simulink model "DemonstratorSimscape_GMM1"  (R2021b)
settings: Solver=ode113  StartTime=0.0  StopTime=t_stop*0+20  FixedStep=1e-4
values from neighbouring files (symbols this model uses):
  brkD = 0    [main.m]
  brkI = 1e4    (= 10000)    [main.m]
  brkP = 1e5    (= 100000)    [main.m]
  d_drm = 0.5*d_drum    [main.m]
  d_shm = 0.4*d_sheave    [main.m]
  DeltaCable0 = 0    [main.m]
  Droop_scaling = 0    [main.m]
  eta_sh = 0.015    [main.m]
  filt_NUM = ones(1,200)*0.005    [main.m]
  g = 9.80665    [main.m]
  Iw = 0.5*(W.i + M.in*GB.r^2)    [main.m]
  Kp_mul = 0.3    [main.m]
  Lc0 = abs((T.ph-L.height-P.d-L.z0)*0.001)    [main.m]
  Ls1 = ((T.ph-0.5*W.pd)/1000)    [main.m]
  Ls2 = ((0.5*(T.s2+P.d)-2*P.d)/1000)    [main.m]
  M = 50e3    (= 50000)    [calcGrav.m]
  phi0_drm = -90    [main.m]
  phi0_shm = -90    [main.m]
  r_sheave = P.d*0.5    [main.m]
  s = tf('s')    [calcGrav.m]
  tau_brk = 0.001    [main.m]
  tau_em = 60e-3    (= 0.06)    [calcGrav.m]    (also in main.m)
  tau_m = tau_w/GB.r    [main.m]
  Tmax = 400e3    (= 400000)    [main.m]
  Tn_mul = 10    [main.m]
  x_drm = 0.7*r_drum    [main.m]
  x_shm = 0.7*r_sheave    [main.m]
  z0 = 0    [calcGrav.m]    (also in main.m = L.z0-P.d*0.5-P.d-P.d-L.height-T.h1-T.h2-32)
undefined symbols (not defined in the file or in its folder): C, CA, Controller_sampleTime, DiscIntNeverNeededParam, GB, L, P, Part, T, VFD_acceleration_model_factor, VFD_Adapt_factor_lower_p1458, VFD_Adapt_factor_upper_p1459, VFD_Curr_limit_var_p0641, VFD_Current_limit_p0640, VFD_Id_setp_total_r1624, VFD_Iq, VFD_Kp_n_basic_p1460, VFD_M, VFD_M_accel_T_smooth_p1517, VFD_M_lim_var_fixS_src_p1551, VFD_M_max_lower_p1521, VFD_M_max_lower_scal_p1525, VFD_M_max_up_mot_scal_p1524, VFD_M_max_upper_p1520, VFD_n_act_T_smooth_p1442, VFD_n_ctr_Kp_n_up_scal_p1461, VFD_n_ctr_Tn_n_up_sca_p1463, VFD_n_ctrl_adapt_Kp_lower_p1456, VFD_n_ctrl_adapt_Kp_upper_p1457, VFD_n_ctrl_Adpt_sig_Kp_p1455, VFD_n_ctrl_Kp_scal_p1466, VFD_n_ctrl_n_lower_p1464, VFD_n_ctrl_n_upper_p1465, VFD_n_ctrl_Tn_n_lower_p1462, VFD_n_limit_neg_p1086, VFD_n_limit_pos_p1083, VFD_n_limit_setp_p1063, VFD_n_max_p1082, VFD_n_set_filt_1_T_p1416, VFD_P_max_gen_p1531, VFD_P_max_mot_p1530, VFD_PU_I_outp_max_r0289, VFD_RFG_ramp_down_time_p1121, VFD_RFG_ramp_up_time_p1120, VFD_RFG_t_RD_scal_p1139, VFD_RFG_t_RU_scal_p1138, VSD, W, X, Y, Z
libraries: sm_lib x248, nesl_utility x128, simulink x49, cstblocks x2, pid_lib x2, slpidlib x2, simulink_extras x2
(part 5 of 11)

== system DemonstratorSimscape_GMM1/Transmission System/Anchor and Load/Sheave_05 ==
  Bending loss : Subsystem  Commented=on
  Gain : Gain  Gain=-1
  Nm : nesl_utility/Simulink-PS Converter  PhysicalDomain=network_engine_domain  SubClassName=ps_input  LeftPortType=input  RightPortType=output  PseudoPeriodic=off  Frequencies=[]  NoiseDistribution=none  NoiseParameters=[]  Unit=1  AffineConversion=off  FilteringAndDerivatives=filter  SimscapeFilterOrder=2  InputFilterTimeConstant=tau_bending  UdotUserProvided=0
      settings: SourceProductBaseCode=PW,SS
  PS>Sim2 : Subsystem
  Pulley 5 : sm_lib/Belts and Cables/Pulley  PitchRadius=P.d*0.5  PitchRadiusUnits=mm  InitialWrapAngleLowerBound=0.0  InitialWrapAngleLowerBoundUnits=deg  SenseWrapAngle=off  SensePulleyAngleA=off  SensePulleyAngleB=off  SenseFleetAngleA=off  SenseFleetAngleB=off
      settings: SourceProductBaseCode=MS
  Revolute Pulley5 : sm_lib/Joints/Revolute Joint  JointMode=Normal  SenseConstraintForce=on  SenseConstraintForceX=off  SenseConstraintForceY=off  SenseConstraintForceZ=off  SenseConstraintTorque=on  SenseConstraintTorqueX=off  SenseConstraintTorqueY=off  SenseConstraintTorqueZ=off  SenseTotalForce=on  SenseTotalForceX=off  SenseTotalForceY=off  SenseTotalForceZ=off  SenseTotalTorque=on  SenseTotalTorqueX=off  SenseTotalTorqueY=off  SenseTotalTorqueZ=off  CompositeWrenchDir=FollowerOnBase  CompositeWrenchFrame=BaseFrame  EquilibriumPosition=0  EquilibriumPositionUnits=deg  SpringStiffness=0  SpringStiffnessUnits=N*m/deg  DampingCoefficient=b_pulley  DampingCoefficientUnits=N*m/(deg/s)  TorqueActuationMode=InputTorque  MotionActuationMode=ComputedMotion  SensePosition=on  SenseVelocity=on  SenseAcceleration=on  SenseTorqueForce=on  SenseLowerLimitTorqueForce=off  SenseUpperLimitTorqueForce=off  LowerLimitSpecify=off  LowerLimitBound=-90  LowerLimitBoundUnits=deg  LowerLimitStiffness=1e4  LowerLimitStiffnessUnits=N*m/deg  LowerLimitDamping=10  LowerLimitDampingUnits=N*m/(deg/s)  LowerLimitTransitionRegionWidth=0.1  LowerLimitTransitionRegionWidthUnits=deg  UpperLimitSpecify=off  UpperLimitBound=90  UpperLimitBoundUnits=deg  UpperLimitStiffness=1e4  UpperLimitStiffnessUnits=N*m/deg  UpperLimitDamping=10  UpperLimitDampingUnits=N*m/(deg/s)  UpperLimitTransitionRegionWidth=0.1  UpperLimitTransitionRegionWidthUnits=deg  PositionTargetSpecify=off  PositionTargetPriority=High  PositionTargetValue=0  PositionTargetValueUnits=deg  VelocityTargetSpecify=off  VelocityTargetPriority=High  VelocityTargetValue=0  VelocityTargetValueUnits=deg/s
  ScopePulley5 : Scope  Commented=on  NumInputPorts=8
  Sheave5 : Subsystem
      mask Display: image('sm_cable_drive_right_angle_pulleyA_IMAGE.png');
  w (rad/s)1 : nesl_utility/PS-Simulink Converter  PhysicalDomain=network_engine_domain  SubClassName=ps_output  LeftPortType=input  RightPortType=output  PseudoPeriodic=off  Frequencies=[]  Unit=rad/s  AffineConversion=on
      settings: SourceProductBaseCode=PW,SS
  ConnS5 : PMIOPort  Side=Right
  WireA : PMIOPort  Port=2  Side=Left
  WireB : PMIOPort  Port=3  Side=Left
  w (rad/s) : Outport
  tag scope: S4=global, w5=global
  wires:
  PS>Sim2/6(Out6) -> ScopePulley5/6
  PS>Sim2/3(Out3) -> ScopePulley5/3
  PS>Sim2/4(Out4) -> ScopePulley5/4
  PS>Sim2/7(Out7) -> ScopePulley5/7
  PS>Sim2/1(Out1) -> ScopePulley5/1
  PS>Sim2/5(Out5) -> ScopePulley5/5
  PS>Sim2/2(Out2) -> ScopePulley5/2
  PS>Sim2/8(Out8) -> ScopePulley5/8
  w (rad/s)1/1 -> Gain/1, w (rad/s)/1
  [S5] -> Bending loss/1(Sin (kN))
  Bending loss/1(dT (Nm)) -> Nm/1
  Bending loss/2(Sout (kN)) -> [S4]
  Gain/1 -> [w5], Bending loss/2(w (deg/s))
  connections:
  w (rad/s)1/LConn1 -- Revolute Pulley5/RConn3 -- PS>Sim2/LConn2
  WireB/RConn1 -- Pulley 5/RConn2
  Revolute Pulley5/RConn4 -- PS>Sim2/LConn3
  Revolute Pulley5/RConn6 -- PS>Sim2/LConn5
  Revolute Pulley5/RConn9 -- PS>Sim2/LConn8
  Revolute Pulley5/RConn7 -- PS>Sim2/LConn6
  Revolute Pulley5/RConn5 -- PS>Sim2/LConn4
  Revolute Pulley5/RConn8 -- PS>Sim2/LConn7
  Revolute Pulley5/RConn2 -- PS>Sim2/LConn1
  Sheave5/RConn1 -- Pulley 5/LConn1
  Sheave5/LConn1 -- Revolute Pulley5/RConn1
  Revolute Pulley5/LConn1 -- ConnS5/RConn1
  Pulley 5/RConn1 -- WireA/RConn1
  Nm/RConn1 -- Revolute Pulley5/LConn2

== system DemonstratorSimscape_GMM1/Transmission System/Anchor and Load/cable mass ==
  "LoadPos [mm] " : Inport
  Add : Sum  Inputs=+-
  CableMass : Scope  Commented=on  NumInputPorts=2
  Constant : Constant  Value=P.up-W.pd*0.5
  Constant4 : Constant  Value=P.up
  Constant5 : Constant  Value=L.height
  Constant6 : Constant  Value=P.d
  Demux : Demux  Outputs=2
  Gain{,4,7,9} (4 alike) : Gain  Gain=CA.mpl
  Gain1 : Gain  Gain=2
  Gain10 : Gain  Gain=0.5
  Gain11 : Gain  Gain=0.5
  Gain12 : Gain  Gain=0.5
  Gain{2,5..6,8} (4 alike) : Gain  Gain=1/1000
  Gain3 : Gain  Gain=4
  Mux : Mux  Inputs=2
  Sum : Sum  Inputs=-+
  Sum1 : Sum  Inputs=+--
  Sum2 : Sum
  Sum3 : Sum
  net cable mass [kg] : Outport  VectorParamsAs1DForOutWhenUnconnected=off
  payout  [m] : Outport  Port=2  VectorParamsAs1DForOutWhenUnconnected=off
  cable mass [kg] : Outport  Port=3  VectorParamsAs1DForOutWhenUnconnected=off
  tag scope: LoadCableMass=global, WinchCableMass=global
  wires:
  Sum1/1 -> Gain3/1
  Constant5/1 -> Sum3/1
  Gain3/1 -> Add/1, Mux/2, Sum2/2, Sum/2
  Gain1/1 -> Add/2, Mux/1, Sum2/1, Sum/1
  Constant6/1 -> Sum3/2
  Constant4/1 -> Sum1/1
  Constant/1 -> Gain1/1
  Sum3/1 -> Sum1/2
  Sum/1 -> Gain5/1
  Gain/1 -> net cable mass [kg]/1
  Gain5/1 -> payout  [m]/1, Gain/1
  "LoadPos [mm] "/1 -> Sum1/3
  Mux/1 -> Gain6/1
  Gain6/1 -> Gain7/1
  Gain7/1 -> Gain10/1
  Sum2/1 -> Gain2/1
  Gain2/1 -> Gain4/1
  Gain4/1 -> cable mass [kg]/1
  Add/1 -> Gain8/1
  Gain8/1 -> Gain9/1
  Gain9/1 -> Gain11/1
  Gain10/1 -> Demux/1, CableMass/1
  Gain11/1 -> CableMass/2
  Gain12/1 -> [LoadCableMass]
  Demux/1 -> [WinchCableMass]
  Demux/2 -> Gain12/1

== system DemonstratorSimscape_GMM1/Transmission System/Roof Pulley Set/ENDS ==
  Belt-Cable End : sm_lib/Belts and Cables/Belt-Cable End
      settings: SourceProductBaseCode=MS
  Belt-Cable End1 : sm_lib/Belts and Cables/Belt-Cable End
      settings: SourceProductBaseCode=MS
  Brick Solid : sm_lib/Body Elements/Brick Solid  GraphicAmbientColor=[0.15 0.15 0.15 1.0]  BasedOnType=Density  BrickDimensions=0.2*[1 1 1]  BrickDimensionUnits=m  CenterOfMass=[0 0 0]  CenterOfMassUnits=m  GraphicDiffuseColor=0.2*[1 1 1]  Density=0  DensityUnits=kg/m^3  DoExposeReferenceFrame=on  GraphicEmissiveColor=[0.0 0.0 0.0 1.0]  ExportEntireGeometry=off  SerializedFrames=<Frames/>  MarkerShape=Sphere  MarkerSize=10  GraphicType=FromGeometry  InertiaType=CalculateFromGeometry  Mass=1  MassUnits=kg  MomentsOfInertia=[1 1 1]  MomentsOfInertiaUnits=kg*m^2  GraphicOpacity=1.0  ProductsOfInertia=[0 0 0]  ProductsOfInertiaUnits=kg*m^2  GraphicShininess=75  GraphicSpecularColor=[0.5 0.5 0.5 1.0]  GraphicVisPropType=SimpleVisualProperties
  Brick Solid1 : sm_lib/Body Elements/Brick Solid  GraphicAmbientColor=[0.15 0.15 0.15 1.0]  BasedOnType=Density  BrickDimensions=0.2*[1 1 1]  BrickDimensionUnits=m  CenterOfMass=[0 0 0]  CenterOfMassUnits=m  GraphicDiffuseColor=0.2*[1 1 1]  Density=0  DensityUnits=kg/m^3  DoExposeReferenceFrame=on  GraphicEmissiveColor=[0.0 0.0 0.0 1.0]  ExportEntireGeometry=off  SerializedFrames=<Frames/>  MarkerShape=Sphere  MarkerSize=10  GraphicType=FromGeometry  InertiaType=CalculateFromGeometry  Mass=1  MassUnits=kg  MomentsOfInertia=[1 1 1]  MomentsOfInertiaUnits=kg*m^2  GraphicOpacity=1.0  ProductsOfInertia=[0 0 0]  ProductsOfInertiaUnits=kg*m^2  GraphicShininess=75  GraphicSpecularColor=[0.5 0.5 0.5 1.0]  GraphicVisPropType=SimpleVisualProperties
  Demux : Demux  Outputs=3
  Demux1 : Demux  Outputs=3
  Ends Tension : Scope  Commented=on
  Mux : Mux
  PS-Simulink Converter : nesl_utility/PS-Simulink Converter  PhysicalDomain=network_engine_domain  SubClassName=ps_output  LeftPortType=input  RightPortType=output  PseudoPeriodic=off  Frequencies=[]  Unit=kN  AffineConversion=off
      settings: SourceProductBaseCode=PW,SS
  PS-Simulink Converter1 : nesl_utility/PS-Simulink Converter  PhysicalDomain=network_engine_domain  SubClassName=ps_output  LeftPortType=input  RightPortType=output  PseudoPeriodic=off  Frequencies=[]  Unit=kN  AffineConversion=off
      settings: SourceProductBaseCode=PW,SS
  Rigid Transform1 : sm_lib/Frames and Transforms/Rigid Transform  TranslationMethod=Cartesian  TranslationStandardOffset=0  TranslationLengthUnit=mm  TranslationStandardAxis=+Z  TranslationCartesianOffset="[-P.Bd*0.5  0 0]"  TranslationROffset=0  TranslationROffsetUnits=m  TranslationZOffset=0  TranslationZOffsetUnits=m  TranslationThetaOffset=0  TranslationThetaOffsetUnits=deg  RotationMethod=None  RotationAngleUnits=deg  RotationStandardAxis=+Z  RotationAngle=0.0  RotationArbitraryAxis=[0 0 1]  FollAlignAxisA=+X  BaseAlignAxisA=+Y  FollAlignAxisB=+Y  BaseAlignAxisB=+Z  RotationSequenceAxes=FollowerAxes  RotationSequence=XYX  RotationSequenceAngles=[0 0 0]  RotationSequenceAnglesUnits=deg  RotationMatrix=[1 0 0; 0 1 0; 0 0 1]
  Rigid Transform3 : sm_lib/Frames and Transforms/Rigid Transform  TranslationMethod=Cartesian  TranslationStandardOffset=0  TranslationLengthUnit=mm  TranslationStandardAxis=+Z  TranslationCartesianOffset="[P.Bd*0.5  0 0]"  TranslationROffset=0  TranslationROffsetUnits=m  TranslationZOffset=0  TranslationZOffsetUnits=m  TranslationThetaOffset=0  TranslationThetaOffsetUnits=deg  RotationMethod=None  RotationAngleUnits=deg  RotationStandardAxis=+Z  RotationAngle=0.0  RotationArbitraryAxis=[0 0 1]  FollAlignAxisA=+X  BaseAlignAxisA=+Y  FollAlignAxisB=+Y  BaseAlignAxisB=+Z  RotationSequenceAxes=FollowerAxes  RotationSequence=XYX  RotationSequenceAngles=[0 0 0]  RotationSequenceAnglesUnits=deg  RotationMatrix=[1 0 0; 0 1 0; 0 0 1]
  Weld Joint : sm_lib/Joints/Weld Joint  JointMode=Normal  SenseConstraintForce=on  SenseConstraintForceX=off  SenseConstraintForceY=off  SenseConstraintForceZ=off  SenseConstraintTorque=off  SenseConstraintTorqueX=off  SenseConstraintTorqueY=off  SenseConstraintTorqueZ=off  SenseTotalForce=off  SenseTotalForceX=off  SenseTotalForceY=off  SenseTotalForceZ=off  SenseTotalTorque=off  SenseTotalTorqueX=off  SenseTotalTorqueY=off  SenseTotalTorqueZ=off  CompositeWrenchDir=BaseOnFollower  CompositeWrenchFrame=FollowerFrame
  Weld Joint1 : sm_lib/Joints/Weld Joint  JointMode=Normal  SenseConstraintForce=on  SenseConstraintForceX=off  SenseConstraintForceY=off  SenseConstraintForceZ=off  SenseConstraintTorque=off  SenseConstraintTorqueX=off  SenseConstraintTorqueY=off  SenseConstraintTorqueZ=off  SenseTotalForce=off  SenseTotalForceX=off  SenseTotalForceY=off  SenseTotalForceZ=off  SenseTotalTorque=off  SenseTotalTorqueX=off  SenseTotalTorqueY=off  SenseTotalTorqueZ=off  CompositeWrenchDir=BaseOnFollower  CompositeWrenchFrame=FollowerFrame
  ConnCentre : PMIOPort  Side=Left
  ConnEndL : PMIOPort  Port=2  Side=Right
  ConnEndR : PMIOPort  Port=3  Side=Right
  wires:
  PS-Simulink Converter/1 -> Demux/1
  PS-Simulink Converter1/1 -> Demux1/1
  Demux1/2 -> Mux/2
  Mux/1 -> Ends Tension/1
  Demux/2 -> Mux/1
  [S3] -> Mux/3
  [S4] -> Mux/4
  connections:
  ConnEndL/RConn1 -- Belt-Cable End1/RConn1
  Rigid Transform3/LConn1 -- Rigid Transform1/LConn1 -- ConnCentre/RConn1
  Weld Joint/RConn1 -- Belt-Cable End/LConn1
  Rigid Transform1/RConn1 -- Brick Solid1/RConn1 -- Weld Joint1/LConn1
  ConnEndR/RConn1 -- Belt-Cable End/RConn1
  Rigid Transform3/RConn1 -- Brick Solid/RConn1 -- Weld Joint/LConn1
  Weld Joint1/RConn1 -- Belt-Cable End1/LConn1
  Weld Joint/RConn2 -- PS-Simulink Converter/LConn1
  PS-Simulink Converter1/LConn1 -- Weld Joint1/RConn2

== system DemonstratorSimscape_GMM1/Transmission System/Roof Pulley Set/Sheave_01 ==
  " " : sm_lib/Frames and Transforms/Rigid Transform  TranslationMethod=Cartesian  TranslationStandardOffset=0  TranslationLengthUnit=mm  TranslationStandardAxis=+Z  TranslationCartesianOffset=[0 -P.d*.25 -P.h]  TranslationROffset=0  TranslationROffsetUnits=m  TranslationZOffset=0  TranslationZOffsetUnits=m  TranslationThetaOffset=0  TranslationThetaOffsetUnits=deg  RotationMethod=ArbitraryAxis  RotationAngleUnits=deg  RotationStandardAxis=+Z  RotationAngle=90  RotationArbitraryAxis=[1 0 0]  FollAlignAxisA=+X  BaseAlignAxisA=+Y  FollAlignAxisB=+Y  BaseAlignAxisB=+Z  RotationSequenceAxes=FollowerAxes  RotationSequence=XYX  RotationSequenceAngles=[0 0 0]  RotationSequenceAnglesUnits=deg  RotationMatrix=[1 0 0; 0 1 0; 0 0 1]
  " 4" : sm_lib/Frames and Transforms/Rigid Transform  TranslationMethod=Cartesian  TranslationStandardOffset=0  TranslationLengthUnit=mm  TranslationStandardAxis=+Z  TranslationCartesianOffset=[0 -P.d*.25 P.h]  TranslationROffset=0  TranslationROffsetUnits=m  TranslationZOffset=0  TranslationZOffsetUnits=m  TranslationThetaOffset=0  TranslationThetaOffsetUnits=deg  RotationMethod=ArbitraryAxis  RotationAngleUnits=deg  RotationStandardAxis=+Z  RotationAngle=90  RotationArbitraryAxis=[1 0 0]  FollAlignAxisA=+X  BaseAlignAxisA=+Y  FollAlignAxisB=+Y  BaseAlignAxisB=+Z  RotationSequenceAxes=FollowerAxes  RotationSequence=XYX  RotationSequenceAngles=[0 0 0]  RotationSequenceAnglesUnits=deg  RotationMatrix=[1 0 0; 0 1 0; 0 0 1]
  Bending loss : Subsystem  Commented=on
  Gain : Gain
  Nm : nesl_utility/Simulink-PS Converter  PhysicalDomain=network_engine_domain  SubClassName=ps_input  LeftPortType=input  RightPortType=output  PseudoPeriodic=off  Frequencies=[]  NoiseDistribution=none  NoiseParameters=[]  Unit=1  AffineConversion=off  FilteringAndDerivatives=filter  SimscapeFilterOrder=2  InputFilterTimeConstant=tau_bending  UdotUserProvided=0
      settings: SourceProductBaseCode=PW,SS
  PS>Sim1 : Subsystem
  Pulley 1 : sm_lib/Belts and Cables/Pulley  PitchRadius=P.d*0.5  PitchRadiusUnits=mm  InitialWrapAngleLowerBound=0.0  InitialWrapAngleLowerBoundUnits=deg  SenseWrapAngle=off  SensePulleyAngleA=off  SensePulleyAngleB=off  SenseFleetAngleA=off  SenseFleetAngleB=off
      settings: SourceProductBaseCode=MS
  Revolute Pulley1 : sm_lib/Joints/Revolute Joint  JointMode=Normal  SenseConstraintForce=on  SenseConstraintForceX=off  SenseConstraintForceY=off  SenseConstraintForceZ=off  SenseConstraintTorque=on  SenseConstraintTorqueX=off  SenseConstraintTorqueY=off  SenseConstraintTorqueZ=off  SenseTotalForce=on  SenseTotalForceX=off  SenseTotalForceY=off  SenseTotalForceZ=off  SenseTotalTorque=on  SenseTotalTorqueX=off  SenseTotalTorqueY=off  SenseTotalTorqueZ=off  CompositeWrenchDir=FollowerOnBase  CompositeWrenchFrame=BaseFrame  EquilibriumPosition=0  EquilibriumPositionUnits=deg  SpringStiffness=0  SpringStiffnessUnits=N*m/deg  DampingCoefficient=b_pulley  DampingCoefficientUnits=N*m/(deg/s)  TorqueActuationMode=InputTorque  MotionActuationMode=ComputedMotion  SensePosition=on  SenseVelocity=on  SenseAcceleration=on  SenseTorqueForce=on  SenseLowerLimitTorqueForce=off  SenseUpperLimitTorqueForce=off  LowerLimitSpecify=off  LowerLimitBound=-90  LowerLimitBoundUnits=deg  LowerLimitStiffness=1e4  LowerLimitStiffnessUnits=N*m/deg  LowerLimitDamping=10  LowerLimitDampingUnits=N*m/(deg/s)  LowerLimitTransitionRegionWidth=0.1  LowerLimitTransitionRegionWidthUnits=deg  UpperLimitSpecify=off  UpperLimitBound=90  UpperLimitBoundUnits=deg  UpperLimitStiffness=1e4  UpperLimitStiffnessUnits=N*m/deg  UpperLimitDamping=10  UpperLimitDampingUnits=N*m/(deg/s)  UpperLimitTransitionRegionWidth=0.1  UpperLimitTransitionRegionWidthUnits=deg  PositionTargetSpecify=off  PositionTargetPriority=High  PositionTargetValue=0  PositionTargetValueUnits=deg  VelocityTargetSpecify=off  VelocityTargetPriority=High  VelocityTargetValue=0  VelocityTargetValueUnits=deg/s
  ScopePulley1 : Scope  Commented=on  NumInputPorts=8
  Sheave1 : Subsystem
      mask Display: image('sm_cable_drive_right_angle_pulleyA_IMAGE.png');
  left face : sm_lib/Body Elements/Brick Solid  GraphicAmbientColor=[0.15 0.15 0.15 1.0]  BasedOnType=Density  BrickDimensions=[P.d P.h P.d*.5]  BrickDimensionUnits=mm  CenterOfMass=[0 0 0]  CenterOfMassUnits=m  GraphicDiffuseColor=[0.6 0.6 0.0]  Density=0  DensityUnits=g/cm^3  DoExposeReferenceFrame=on  GraphicEmissiveColor=[0.0 0.0 0.0 1.0]  ExportEntireGeometry=off  SerializedFrames=<Frames/>  MarkerShape=Sphere  MarkerSize=10  GraphicType=FromGeometry  InertiaType=CalculateFromGeometry  Mass=1  MassUnits=kg  MomentsOfInertia=[1 1 1]  MomentsOfInertiaUnits=kg*m^2  GraphicOpacity=c.opac  ProductsOfInertia=[0 0 0]  ProductsOfInertiaUnits=kg*m^2  GraphicShininess=75  GraphicSpecularColor=[0.5 0.5 0.5 1.0]  GraphicVisPropType=SimpleVisualProperties
  right face : sm_lib/Body Elements/Brick Solid  GraphicAmbientColor=[0.15 0.15 0.15 1.0]  BasedOnType=Density  BrickDimensions=[P.d P.h P.d*.5]  BrickDimensionUnits=mm  CenterOfMass=[0 0 0]  CenterOfMassUnits=m  GraphicDiffuseColor=[0.6 0.6 0.0]  Density=0  DensityUnits=g/cm^3  DoExposeReferenceFrame=on  GraphicEmissiveColor=[0.0 0.0 0.0 1.0]  ExportEntireGeometry=off  SerializedFrames=<Frames/>  MarkerShape=Sphere  MarkerSize=10  GraphicType=FromGeometry  InertiaType=CalculateFromGeometry  Mass=1  MassUnits=kg  MomentsOfInertia=[1 1 1]  MomentsOfInertiaUnits=kg*m^2  GraphicOpacity=1.0  ProductsOfInertia=[0 0 0]  ProductsOfInertiaUnits=kg*m^2  GraphicShininess=75  GraphicSpecularColor=[0.5 0.5 0.5 1.0]  GraphicVisPropType=SimpleVisualProperties
  w (rad/s)1 : nesl_utility/PS-Simulink Converter  PhysicalDomain=network_engine_domain  SubClassName=ps_output  LeftPortType=input  RightPortType=output  PseudoPeriodic=off  Frequencies=[]  Unit=rad/s  AffineConversion=off
      settings: SourceProductBaseCode=PW,SS
  WireA : PMIOPort  Side=Right
  Conn1 : PMIOPort  Port=2  Side=Left
  WireB : PMIOPort  Port=3  Side=Right
  w (rad/s) : Outport
  tag scope: S1=global, w1=global
  wires:
  w (rad/s)1/1 -> [w1], Gain/1, w (rad/s)/1
  PS>Sim1/5(Out5) -> ScopePulley1/5
  PS>Sim1/8(Out8) -> ScopePulley1/8
  PS>Sim1/2(Out2) -> ScopePulley1/2
  PS>Sim1/1(Out1) -> ScopePulley1/1
  PS>Sim1/3(Out3) -> ScopePulley1/3
  PS>Sim1/7(Out7) -> ScopePulley1/7
  PS>Sim1/4(Out4) -> ScopePulley1/4
  PS>Sim1/6(Out6) -> ScopePulley1/6
  Bending loss/1(dT (Nm)) -> Nm/1
  Bending loss/2(Sout (kN)) -> [S1]
  [S0] -> Bending loss/1(Sin (kN))
  Gain/1 -> Bending loss/2(w (deg/s))
  connections:
  Pulley 1/RConn1 -- WireA/RConn1
  Sheave1/RConn1 -- Pulley 1/LConn1
  Pulley 1/RConn2 -- WireB/RConn1
  PS>Sim1/LConn2 -- Revolute Pulley1/RConn3 -- w (rad/s)1/LConn1
  " 4"/LConn1 -- " "/LConn1 -- Conn1/RConn1 -- Revolute Pulley1/LConn1
  Revolute Pulley1/RConn6 -- PS>Sim1/LConn5
  Revolute Pulley1/RConn2 -- PS>Sim1/LConn1
  Sheave1/LConn1 -- Revolute Pulley1/RConn1
  " "/RConn1 -- right face/RConn1
  Revolute Pulley1/RConn4 -- PS>Sim1/LConn3
  Revolute Pulley1/RConn9 -- PS>Sim1/LConn8
  Revolute Pulley1/RConn8 -- PS>Sim1/LConn7
  Revolute Pulley1/RConn5 -- PS>Sim1/LConn4
  Revolute Pulley1/RConn7 -- PS>Sim1/LConn6
  " 4"/RConn1 -- left face/RConn1
  Nm/RConn1 -- Revolute Pulley1/LConn2

== system DemonstratorSimscape_GMM1/Transmission System/Roof Pulley Set/Sheave_02 ==
  " " : sm_lib/Frames and Transforms/Rigid Transform  TranslationMethod=Cartesian  TranslationStandardOffset=0  TranslationLengthUnit=mm  TranslationStandardAxis=+Z  TranslationCartesianOffset=[0 -P.d*.25 -P.h]  TranslationROffset=0  TranslationROffsetUnits=m  TranslationZOffset=0  TranslationZOffsetUnits=m  TranslationThetaOffset=0  TranslationThetaOffsetUnits=deg  RotationMethod=ArbitraryAxis  RotationAngleUnits=deg  RotationStandardAxis=+Z  RotationAngle=90  RotationArbitraryAxis=[1 0 0]  FollAlignAxisA=+X  BaseAlignAxisA=+Y  FollAlignAxisB=+Y  BaseAlignAxisB=+Z  RotationSequenceAxes=FollowerAxes  RotationSequence=XYX  RotationSequenceAngles=[0 0 0]  RotationSequenceAnglesUnits=deg  RotationMatrix=[1 0 0; 0 1 0; 0 0 1]
  " 4" : sm_lib/Frames and Transforms/Rigid Transform  TranslationMethod=Cartesian  TranslationStandardOffset=0  TranslationLengthUnit=mm  TranslationStandardAxis=+Z  TranslationCartesianOffset=[0 -P.d*.25 P.h]  TranslationROffset=0  TranslationROffsetUnits=m  TranslationZOffset=0  TranslationZOffsetUnits=m  TranslationThetaOffset=0  TranslationThetaOffsetUnits=deg  RotationMethod=ArbitraryAxis  RotationAngleUnits=deg  RotationStandardAxis=+Z  RotationAngle=90  RotationArbitraryAxis=[1 0 0]  FollAlignAxisA=+X  BaseAlignAxisA=+Y  FollAlignAxisB=+Y  BaseAlignAxisB=+Z  RotationSequenceAxes=FollowerAxes  RotationSequence=XYX  RotationSequenceAngles=[0 0 0]  RotationSequenceAnglesUnits=deg  RotationMatrix=[1 0 0; 0 1 0; 0 0 1]
  Bending loss : Subsystem  Commented=on
  Constant : Constant  Value=g*1000
  Demux : Demux  Outputs=3
  Divide : Product  Inputs=*/
  Gain : Gain
  Gain1 : Gain  Gain=-2
  Nm : nesl_utility/Simulink-PS Converter  PhysicalDomain=network_engine_domain  SubClassName=ps_input  LeftPortType=input  RightPortType=output  PseudoPeriodic=off  Frequencies=[]  NoiseDistribution=none  NoiseParameters=[]  Unit=1  AffineConversion=off  FilteringAndDerivatives=filter  SimscapeFilterOrder=2  InputFilterTimeConstant=tau_bending  UdotUserProvided=0
      settings: SourceProductBaseCode=PW,SS
  PS>Sim1 : Subsystem
  Pulley 2 : sm_lib/Belts and Cables/Pulley  PitchRadius=P.d*0.5  PitchRadiusUnits=mm  InitialWrapAngleLowerBound=0.0  InitialWrapAngleLowerBoundUnits=deg  SenseWrapAngle=off  SensePulleyAngleA=off  SensePulleyAngleB=off  SenseFleetAngleA=off  SenseFleetAngleB=off
      settings: SourceProductBaseCode=MS
  Revolute Pulley2 : sm_lib/Joints/Revolute Joint  JointMode=Normal  SenseConstraintForce=on  SenseConstraintForceX=off  SenseConstraintForceY=off  SenseConstraintForceZ=off  SenseConstraintTorque=on  SenseConstraintTorqueX=off  SenseConstraintTorqueY=off  SenseConstraintTorqueZ=off  SenseTotalForce=on  SenseTotalForceX=off  SenseTotalForceY=off  SenseTotalForceZ=off  SenseTotalTorque=on  SenseTotalTorqueX=off  SenseTotalTorqueY=off  SenseTotalTorqueZ=off  CompositeWrenchDir=FollowerOnBase  CompositeWrenchFrame=BaseFrame  EquilibriumPosition=0  EquilibriumPositionUnits=deg  SpringStiffness=0  SpringStiffnessUnits=N*m/deg  DampingCoefficient=b_pulley  DampingCoefficientUnits=N*m/(deg/s)  TorqueActuationMode=InputTorque  MotionActuationMode=ComputedMotion  SensePosition=on  SenseVelocity=on  SenseAcceleration=on  SenseTorqueForce=on  SenseLowerLimitTorqueForce=off  SenseUpperLimitTorqueForce=off  LowerLimitSpecify=off  LowerLimitBound=-90  LowerLimitBoundUnits=deg  LowerLimitStiffness=1e4  LowerLimitStiffnessUnits=N*m/deg  LowerLimitDamping=10  LowerLimitDampingUnits=N*m/(deg/s)  LowerLimitTransitionRegionWidth=0.1  LowerLimitTransitionRegionWidthUnits=deg  UpperLimitSpecify=off  UpperLimitBound=90  UpperLimitBoundUnits=deg  UpperLimitStiffness=1e4  UpperLimitStiffnessUnits=N*m/deg  UpperLimitDamping=10  UpperLimitDampingUnits=N*m/(deg/s)  UpperLimitTransitionRegionWidth=0.1  UpperLimitTransitionRegionWidthUnits=deg  PositionTargetSpecify=off  PositionTargetPriority=High  PositionTargetValue=0  PositionTargetValueUnits=deg  VelocityTargetSpecify=off  VelocityTargetPriority=High  VelocityTargetValue=0  VelocityTargetValueUnits=deg/s
  ScopePulley2 : Scope  Commented=on  NumInputPorts=8
  Sheave2 : Subsystem
      mask Display: image('sm_cable_drive_right_angle_pulleyA_IMAGE.png');
  left face : sm_lib/Body Elements/Brick Solid  GraphicAmbientColor=[0.15 0.15 0.15 1.0]  BasedOnType=Density  BrickDimensions=[P.d P.h P.d*.5]  BrickDimensionUnits=mm  CenterOfMass=[0 0 0]  CenterOfMassUnits=m  GraphicDiffuseColor=[0.6 0.6 0.0]  Density=0  DensityUnits=g/cm^3  DoExposeReferenceFrame=on  GraphicEmissiveColor=[0.0 0.0 0.0 1.0]  ExportEntireGeometry=off  SerializedFrames=<Frames/>  MarkerShape=Sphere  MarkerSize=10  GraphicType=FromGeometry  InertiaType=CalculateFromGeometry  Mass=1  MassUnits=kg  MomentsOfInertia=[1 1 1]  MomentsOfInertiaUnits=kg*m^2  GraphicOpacity=c.opac  ProductsOfInertia=[0 0 0]  ProductsOfInertiaUnits=kg*m^2  GraphicShininess=75  GraphicSpecularColor=[0.5 0.5 0.5 1.0]  GraphicVisPropType=SimpleVisualProperties
  right face : sm_lib/Body Elements/Brick Solid  GraphicAmbientColor=[0.15 0.15 0.15 1.0]  BasedOnType=Density  BrickDimensions=[P.d P.h P.d*.5]  BrickDimensionUnits=mm  CenterOfMass=[0 0 0]  CenterOfMassUnits=m  GraphicDiffuseColor=[0.6 0.6 0.0]  Density=0  DensityUnits=g/cm^3  DoExposeReferenceFrame=on  GraphicEmissiveColor=[0.0 0.0 0.0 1.0]  ExportEntireGeometry=off  SerializedFrames=<Frames/>  MarkerShape=Sphere  MarkerSize=10  GraphicType=FromGeometry  InertiaType=CalculateFromGeometry  Mass=1  MassUnits=kg  MomentsOfInertia=[1 1 1]  MomentsOfInertiaUnits=kg*m^2  GraphicOpacity=1.0  ProductsOfInertia=[0 0 0]  ProductsOfInertiaUnits=kg*m^2  GraphicShininess=75  GraphicSpecularColor=[0.5 0.5 0.5 1.0]  GraphicVisPropType=SimpleVisualProperties
  w (rad/s)1 : nesl_utility/PS-Simulink Converter  PhysicalDomain=network_engine_domain  SubClassName=ps_output  LeftPortType=input  RightPortType=output  PseudoPeriodic=off  Frequencies=[]  Unit=rad/s  AffineConversion=off
      settings: SourceProductBaseCode=PW,SS
  Conn1 : PMIOPort  Side=Left
  WireA : PMIOPort  Port=2  Side=Right
  WireB : PMIOPort  Port=3  Side=Right
  w (rad/s) : Outport
  tag scope: PinLoad_L_tonne=global, S2=global, w2=global
  wires:
  PS>Sim1/7(Out7) -> ScopePulley2/7
  w (rad/s)1/1 -> w (rad/s)/1, [w2], Gain/1
  PS>Sim1/2(Out2) -> ScopePulley2/2
  PS>Sim1/3(Out3) -> ScopePulley2/3
  PS>Sim1/8(Out8) -> ScopePulley2/8
  PS>Sim1/1(Out1) -> ScopePulley2/1
  PS>Sim1/5(Out5) -> Demux/1, ScopePulley2/5
  PS>Sim1/4(Out4) -> ScopePulley2/4
  PS>Sim1/6(Out6) -> ScopePulley2/6
  [S1] -> Bending loss/1(Sin (kN))
  Bending loss/2(Sout (kN)) -> [S2]
  Gain/1 -> Bending loss/2(w (deg/s))
  Bending loss/1(dT (Nm)) -> Nm/1
  Divide/1 -> [PinLoad_L_tonne]
  Gain1/1 -> Divide/1
  Constant/1 -> Divide/2
  Demux/2 -> Gain1/1
  connections:
  Sheave2/RConn1 -- Pulley 2/LConn1
  Pulley 2/RConn1 -- WireA/RConn1
  WireB/RConn1 -- Pulley 2/RConn2
  Revolute Pulley2/LConn1 -- Conn1/RConn1 -- " "/LConn1 -- " 4"/LConn1
  PS>Sim1/LConn2 -- w (rad/s)1/LConn1 -- Revolute Pulley2/RConn3
  Sheave2/LConn1 -- Revolute Pulley2/RConn1
  " "/RConn1 -- right face/RConn1
  Revolute Pulley2/RConn8 -- PS>Sim1/LConn7
  Revolute Pulley2/RConn6 -- PS>Sim1/LConn5
  " 4"/RConn1 -- left face/RConn1
  Revolute Pulley2/RConn2 -- PS>Sim1/LConn1
  Revolute Pulley2/RConn7 -- PS>Sim1/LConn6
  Revolute Pulley2/RConn5 -- PS>Sim1/LConn4
  Revolute Pulley2/RConn4 -- PS>Sim1/LConn3
  Revolute Pulley2/RConn9 -- PS>Sim1/LConn8
  Nm/RConn1 -- Revolute Pulley2/LConn2

== system DemonstratorSimscape_GMM1/Transmission System/Roof Pulley Set/Sheave_04 ==
  " " : sm_lib/Frames and Transforms/Rigid Transform  TranslationMethod=Cartesian  TranslationStandardOffset=0  TranslationLengthUnit=mm  TranslationStandardAxis=+Z  TranslationCartesianOffset=[0 -P.Bd*.25 -P.h]  TranslationROffset=0  TranslationROffsetUnits=m  TranslationZOffset=0  TranslationZOffsetUnits=m  TranslationThetaOffset=0  TranslationThetaOffsetUnits=deg  RotationMethod=ArbitraryAxis  RotationAngleUnits=deg  RotationStandardAxis=+Z  RotationAngle=90  RotationArbitraryAxis=[1 0 0]  FollAlignAxisA=+X  BaseAlignAxisA=+Y  FollAlignAxisB=+Y  BaseAlignAxisB=+Z  RotationSequenceAxes=FollowerAxes  RotationSequence=XYX  RotationSequenceAngles=[0 0 0]  RotationSequenceAnglesUnits=deg  RotationMatrix=[1 0 0; 0 1 0; 0 0 1]
  " 4" : sm_lib/Frames and Transforms/Rigid Transform  TranslationMethod=Cartesian  TranslationStandardOffset=0  TranslationLengthUnit=mm  TranslationStandardAxis=+Z  TranslationCartesianOffset=[0 -P.Bd*.25 P.h]  TranslationROffset=0  TranslationROffsetUnits=m  TranslationZOffset=0  TranslationZOffsetUnits=m  TranslationThetaOffset=0  TranslationThetaOffsetUnits=deg  RotationMethod=ArbitraryAxis  RotationAngleUnits=deg  RotationStandardAxis=+Z  RotationAngle=90  RotationArbitraryAxis=[1 0 0]  FollAlignAxisA=+X  BaseAlignAxisA=+Y  FollAlignAxisB=+Y  BaseAlignAxisB=+Z  RotationSequenceAxes=FollowerAxes  RotationSequence=XYX  RotationSequenceAngles=[0 0 0]  RotationSequenceAnglesUnits=deg  RotationMatrix=[1 0 0; 0 1 0; 0 0 1]
  PS>Sim1 : Subsystem
  Pulley 5 : sm_lib/Belts and Cables/Pulley  PitchRadius=P.Bd*0.5  PitchRadiusUnits=mm  InitialWrapAngleLowerBound=0.0  InitialWrapAngleLowerBoundUnits=deg  SenseWrapAngle=off  SensePulleyAngleA=off  SensePulleyAngleB=off  SenseFleetAngleA=off  SenseFleetAngleB=off
      settings: SourceProductBaseCode=MS
  Pulley rught red2 : Subsystem
      mask Display: image('sm_cable_drive_right_angle_pulleyA_IMAGE.png');
  Revolute Pulley5 : sm_lib/Joints/Revolute Joint  JointMode=Normal  SenseConstraintForce=on  SenseConstraintForceX=off  SenseConstraintForceY=off  SenseConstraintForceZ=off  SenseConstraintTorque=on  SenseConstraintTorqueX=off  SenseConstraintTorqueY=off  SenseConstraintTorqueZ=off  SenseTotalForce=on  SenseTotalForceX=off  SenseTotalForceY=off  SenseTotalForceZ=off  SenseTotalTorque=on  SenseTotalTorqueX=off  SenseTotalTorqueY=off  SenseTotalTorqueZ=off  CompositeWrenchDir=FollowerOnBase  CompositeWrenchFrame=BaseFrame  EquilibriumPosition=0  EquilibriumPositionUnits=deg  SpringStiffness=0  SpringStiffnessUnits=N*m/deg  DampingCoefficient=b_pulley  DampingCoefficientUnits=N*m/(deg/s)  TorqueActuationMode=NoTorque  MotionActuationMode=ComputedMotion  SensePosition=on  SenseVelocity=on  SenseAcceleration=on  SenseTorqueForce=on  SenseLowerLimitTorqueForce=off  SenseUpperLimitTorqueForce=off  LowerLimitSpecify=off  LowerLimitBound=-90  LowerLimitBoundUnits=deg  LowerLimitStiffness=1e4  LowerLimitStiffnessUnits=N*m/deg  LowerLimitDamping=10  LowerLimitDampingUnits=N*m/(deg/s)  LowerLimitTransitionRegionWidth=0.1  LowerLimitTransitionRegionWidthUnits=deg  UpperLimitSpecify=off  UpperLimitBound=90  UpperLimitBoundUnits=deg  UpperLimitStiffness=1e4  UpperLimitStiffnessUnits=N*m/deg  UpperLimitDamping=10  UpperLimitDampingUnits=N*m/(deg/s)  UpperLimitTransitionRegionWidth=0.1  UpperLimitTransitionRegionWidthUnits=deg  PositionTargetSpecify=off  PositionTargetPriority=High  PositionTargetValue=0  PositionTargetValueUnits=deg  VelocityTargetSpecify=off  VelocityTargetPriority=High  VelocityTargetValue=0  VelocityTargetValueUnits=deg/s
  ScopePulley5 : Scope  Commented=on  NumInputPorts=8
  Solid : sm_lib/Body Elements/Spherical Solid  GraphicAmbientColor=[0.15 0.15 0.15 1.0]  BasedOnType=Mass  CenterOfMass=[0 0 0]  CenterOfMassUnits=m  GraphicDiffuseColor=[0.5 0.5 0.5]  Density=1000  DensityUnits=kg/m^3  DoExposeReferenceFrame=on  GraphicEmissiveColor=[0.0 0.0 0.0 1.0]  ExportEntireGeometry=off  SerializedExposedGeometries=<ExposedGeometries/>  SerializedFrames=<Frames/>  MarkerShape=Sphere  MarkerSize=10  GraphicType=FromGeometry  InertiaType=CalculateFromGeometry  Mass=0.01  MassUnits=kg  MomentsOfInertia=[1 1 1]  MomentsOfInertiaUnits=kg*m^2  GraphicOpacity=1.0  ProductsOfInertia=[0 0 0]  ProductsOfInertiaUnits=kg*m^2  GraphicShininess=75  GraphicSpecularColor=[0.5 0.5 0.5 1.0]  SphereRadius=0.00001  SphereRadiusUnits=m  GraphicVisPropType=SimpleVisualProperties
  left face : sm_lib/Body Elements/Brick Solid  GraphicAmbientColor=[0.15 0.15 0.15 1.0]  BasedOnType=Density  BrickDimensions=[P.Bd P.h P.Bd*.5]  BrickDimensionUnits=mm  CenterOfMass=[0 0 0]  CenterOfMassUnits=m  GraphicDiffuseColor=[0.6 0.6 0.0]  Density=0  DensityUnits=g/cm^3  DoExposeReferenceFrame=on  GraphicEmissiveColor=[0.0 0.0 0.0 1.0]  ExportEntireGeometry=off  SerializedFrames=<Frames/>  MarkerShape=Sphere  MarkerSize=10  GraphicType=FromGeometry  InertiaType=CalculateFromGeometry  Mass=1  MassUnits=kg  MomentsOfInertia=[1 1 1]  MomentsOfInertiaUnits=kg*m^2  GraphicOpacity=c.opac  ProductsOfInertia=[0 0 0]  ProductsOfInertiaUnits=kg*m^2  GraphicShininess=75  GraphicSpecularColor=[0.5 0.5 0.5 1.0]  GraphicVisPropType=SimpleVisualProperties
  right face : sm_lib/Body Elements/Brick Solid  GraphicAmbientColor=[0.15 0.15 0.15 1.0]  BasedOnType=Density  BrickDimensions=[P.Bd P.h P.Bd*.5]  BrickDimensionUnits=mm  CenterOfMass=[0 0 0]  CenterOfMassUnits=m  GraphicDiffuseColor=[0.6 0.6 0.0]  Density=0  DensityUnits=g/cm^3  DoExposeReferenceFrame=on  GraphicEmissiveColor=[0.0 0.0 0.0 1.0]  ExportEntireGeometry=off  SerializedFrames=<Frames/>  MarkerShape=Sphere  MarkerSize=10  GraphicType=FromGeometry  InertiaType=CalculateFromGeometry  Mass=1  MassUnits=kg  MomentsOfInertia=[1 1 1]  MomentsOfInertiaUnits=kg*m^2  GraphicOpacity=1.0  ProductsOfInertia=[0 0 0]  ProductsOfInertiaUnits=kg*m^2  GraphicShininess=75  GraphicSpecularColor=[0.5 0.5 0.5 1.0]  GraphicVisPropType=SimpleVisualProperties
  w (rad/s) : nesl_utility/PS-Simulink Converter  PhysicalDomain=network_engine_domain  SubClassName=ps_output  LeftPortType=input  RightPortType=output  PseudoPeriodic=off  Frequencies=[]  Unit=rad/s  AffineConversion=off
      settings: SourceProductBaseCode=PW,SS
  B : PMIOPort  Side=Left
  WireB : PMIOPort  Port=2  Side=Right
  WireA : PMIOPort  Port=3  Side=Right
  w5 : Outport  VectorParamsAs1DForOutWhenUnconnected=off
  wires:
  PS>Sim1/6(Out6) -> ScopePulley5/6
  PS>Sim1/3(Out3) -> ScopePulley5/3
  PS>Sim1/2(Out2) -> ScopePulley5/2
  PS>Sim1/1(Out1) -> ScopePulley5/1
  PS>Sim1/8(Out8) -> ScopePulley5/8
  PS>Sim1/7(Out7) -> ScopePulley5/7
  PS>Sim1/4(Out4) -> ScopePulley5/4
  PS>Sim1/5(Out5) -> ScopePulley5/5
  w (rad/s)/1 -> w5/1
  connections:
  " "/LConn1 -- B/RConn1 -- Revolute Pulley5/LConn1 -- " 4"/LConn1
  Solid/RConn1 -- Revolute Pulley5/RConn1 -- Pulley rught red2/LConn1
  Revolute Pulley5/RConn6 -- PS>Sim1/LConn5
  Revolute Pulley5/RConn4 -- PS>Sim1/LConn3
  Revolute Pulley5/RConn7 -- PS>Sim1/LConn6
  Revolute Pulley5/RConn5 -- PS>Sim1/LConn4
  Revolute Pulley5/RConn9 -- PS>Sim1/LConn8
  Revolute Pulley5/RConn8 -- PS>Sim1/LConn7
  Revolute Pulley5/RConn3 -- w (rad/s)/LConn1 -- PS>Sim1/LConn2
  Revolute Pulley5/RConn2 -- PS>Sim1/LConn1
  " 4"/RConn1 -- left face/RConn1
  " "/RConn1 -- right face/RConn1
  WireB/RConn1 -- Pulley 5/RConn2
  Pulley rught red2/RConn1 -- Pulley 5/LConn1
  WireA/RConn1 -- Pulley 5/RConn1

== system DemonstratorSimscape_GMM1/Transmission System/Roof Pulley Set/Sheave_06 ==
  " " : sm_lib/Frames and Transforms/Rigid Transform  TranslationMethod=Cartesian  TranslationStandardOffset=0  TranslationLengthUnit=mm  TranslationStandardAxis=+Z  TranslationCartesianOffset=[0 -P.d*.25 -P.h]  TranslationROffset=0  TranslationROffsetUnits=m  TranslationZOffset=0  TranslationZOffsetUnits=m  TranslationThetaOffset=0  TranslationThetaOffsetUnits=deg  RotationMethod=ArbitraryAxis  RotationAngleUnits=deg  RotationStandardAxis=+Z  RotationAngle=90  RotationArbitraryAxis=[1 0 0]  FollAlignAxisA=+X  BaseAlignAxisA=+Y  FollAlignAxisB=+Y  BaseAlignAxisB=+Z  RotationSequenceAxes=FollowerAxes  RotationSequence=XYX  RotationSequenceAngles=[0 0 0]  RotationSequenceAnglesUnits=deg  RotationMatrix=[1 0 0; 0 1 0; 0 0 1]
  " 4" : sm_lib/Frames and Transforms/Rigid Transform  TranslationMethod=Cartesian  TranslationStandardOffset=0  TranslationLengthUnit=mm  TranslationStandardAxis=+Z  TranslationCartesianOffset=[0 -P.d*.25 P.h]  TranslationROffset=0  TranslationROffsetUnits=m  TranslationZOffset=0  TranslationZOffsetUnits=m  TranslationThetaOffset=0  TranslationThetaOffsetUnits=deg  RotationMethod=ArbitraryAxis  RotationAngleUnits=deg  RotationStandardAxis=+Z  RotationAngle=90  RotationArbitraryAxis=[1 0 0]  FollAlignAxisA=+X  BaseAlignAxisA=+Y  FollAlignAxisB=+Y  BaseAlignAxisB=+Z  RotationSequenceAxes=FollowerAxes  RotationSequence=XYX  RotationSequenceAngles=[0 0 0]  RotationSequenceAnglesUnits=deg  RotationMatrix=[1 0 0; 0 1 0; 0 0 1]
  Bending loss : Subsystem  Commented=on
  Constant : Constant  Value=g*1000
  Demux : Demux  Outputs=3
  Divide : Product  Inputs=*/
  Gain : Gain
  Gain1 : Gain  Gain=-2
  Nm : nesl_utility/Simulink-PS Converter  PhysicalDomain=network_engine_domain  SubClassName=ps_input  LeftPortType=input  RightPortType=output  PseudoPeriodic=off  Frequencies=[]  NoiseDistribution=none  NoiseParameters=[]  Unit=1  AffineConversion=off  FilteringAndDerivatives=filter  SimscapeFilterOrder=2  InputFilterTimeConstant=tau_bending  UdotUserProvided=0
      settings: SourceProductBaseCode=PW,SS
  PS>Sim1 : Subsystem
  Pulley 6 : sm_lib/Belts and Cables/Pulley  PitchRadius=P.d*0.5  PitchRadiusUnits=mm  InitialWrapAngleLowerBound=0.0  InitialWrapAngleLowerBoundUnits=deg  SenseWrapAngle=off  SensePulleyAngleA=off  SensePulleyAngleB=off  SenseFleetAngleA=off  SenseFleetAngleB=off
      settings: SourceProductBaseCode=MS
  Revolute Pulley6 : sm_lib/Joints/Revolute Joint  JointMode=Normal  SenseConstraintForce=on  SenseConstraintForceX=off  SenseConstraintForceY=off  SenseConstraintForceZ=off  SenseConstraintTorque=on  SenseConstraintTorqueX=off  SenseConstraintTorqueY=off  SenseConstraintTorqueZ=off  SenseTotalForce=on  SenseTotalForceX=off  SenseTotalForceY=off  SenseTotalForceZ=off  SenseTotalTorque=on  SenseTotalTorqueX=off  SenseTotalTorqueY=off  SenseTotalTorqueZ=off  CompositeWrenchDir=FollowerOnBase  CompositeWrenchFrame=BaseFrame  EquilibriumPosition=0  EquilibriumPositionUnits=deg  SpringStiffness=0  SpringStiffnessUnits=N*m/deg  DampingCoefficient=b_pulley  DampingCoefficientUnits=N*m/(deg/s)  TorqueActuationMode=InputTorque  MotionActuationMode=ComputedMotion  SensePosition=on  SenseVelocity=on  SenseAcceleration=on  SenseTorqueForce=on  SenseLowerLimitTorqueForce=off  SenseUpperLimitTorqueForce=off  LowerLimitSpecify=off  LowerLimitBound=-90  LowerLimitBoundUnits=deg  LowerLimitStiffness=1e4  LowerLimitStiffnessUnits=N*m/deg  LowerLimitDamping=10  LowerLimitDampingUnits=N*m/(deg/s)  LowerLimitTransitionRegionWidth=0.1  LowerLimitTransitionRegionWidthUnits=deg  UpperLimitSpecify=off  UpperLimitBound=90  UpperLimitBoundUnits=deg  UpperLimitStiffness=1e4  UpperLimitStiffnessUnits=N*m/deg  UpperLimitDamping=10  UpperLimitDampingUnits=N*m/(deg/s)  UpperLimitTransitionRegionWidth=0.1  UpperLimitTransitionRegionWidthUnits=deg  PositionTargetSpecify=off  PositionTargetPriority=High  PositionTargetValue=0  PositionTargetValueUnits=deg  VelocityTargetSpecify=off  VelocityTargetPriority=High  VelocityTargetValue=0  VelocityTargetValueUnits=deg/s
  ScopePulley6 : Scope  Commented=on  NumInputPorts=8
  Sheave6 : Subsystem
      mask Display: image('sm_cable_drive_right_angle_pulleyA_IMAGE.png');
  left face : sm_lib/Body Elements/Brick Solid  GraphicAmbientColor=[0.15 0.15 0.15 1.0]  BasedOnType=Density  BrickDimensions=[P.d P.h P.d*.5]  BrickDimensionUnits=mm  CenterOfMass=[0 0 0]  CenterOfMassUnits=m  GraphicDiffuseColor=[0.6 0.6 0.0]  Density=0  DensityUnits=g/cm^3  DoExposeReferenceFrame=on  GraphicEmissiveColor=[0.0 0.0 0.0 1.0]  ExportEntireGeometry=off  SerializedFrames=<Frames/>  MarkerShape=Sphere  MarkerSize=10  GraphicType=FromGeometry  InertiaType=CalculateFromGeometry  Mass=1  MassUnits=kg  MomentsOfInertia=[1 1 1]  MomentsOfInertiaUnits=kg*m^2  GraphicOpacity=c.opac  ProductsOfInertia=[0 0 0]  ProductsOfInertiaUnits=kg*m^2  GraphicShininess=75  GraphicSpecularColor=[0.5 0.5 0.5 1.0]  GraphicVisPropType=SimpleVisualProperties
  right face : sm_lib/Body Elements/Brick Solid  GraphicAmbientColor=[0.15 0.15 0.15 1.0]  BasedOnType=Density  BrickDimensions=[P.d P.h P.d*.5]  BrickDimensionUnits=mm  CenterOfMass=[0 0 0]  CenterOfMassUnits=m  GraphicDiffuseColor=[0.6 0.6 0.0]  Density=0  DensityUnits=g/cm^3  DoExposeReferenceFrame=on  GraphicEmissiveColor=[0.0 0.0 0.0 1.0]  ExportEntireGeometry=off  SerializedFrames=<Frames/>  MarkerShape=Sphere  MarkerSize=10  GraphicType=FromGeometry  InertiaType=CalculateFromGeometry  Mass=1  MassUnits=kg  MomentsOfInertia=[1 1 1]  MomentsOfInertiaUnits=kg*m^2  GraphicOpacity=1.0  ProductsOfInertia=[0 0 0]  ProductsOfInertiaUnits=kg*m^2  GraphicShininess=75  GraphicSpecularColor=[0.5 0.5 0.5 1.0]  GraphicVisPropType=SimpleVisualProperties
  w (rad/s)1 : nesl_utility/PS-Simulink Converter  PhysicalDomain=network_engine_domain  SubClassName=ps_output  LeftPortType=input  RightPortType=output  PseudoPeriodic=off  Frequencies=[]  Unit=rad/s  AffineConversion=off
      settings: SourceProductBaseCode=PW,SS
  WireA : PMIOPort  Side=Right
  Conn2 : PMIOPort  Port=2  Side=Left
  WireB : PMIOPort  Port=3  Side=Right
  w (rad/s) : Outport
  tag scope: PinLoad_R_tonne=global, S5=global, w6=global
  wires:
  [S6] -> Bending loss/1(Sin (kN))
  Bending loss/1(dT (Nm)) -> Nm/1
  Bending loss/2(Sout (kN)) -> [S5]
  Gain/1 -> Bending loss/2(w (deg/s))
  w (rad/s)1/1 -> Gain/1, [w6], w (rad/s)/1
  PS>Sim1/7(Out7) -> ScopePulley6/7
  PS>Sim1/4(Out4) -> ScopePulley6/4
  PS>Sim1/5(Out5) -> Demux/1, ScopePulley6/5
  PS>Sim1/1(Out1) -> ScopePulley6/1
  PS>Sim1/8(Out8) -> ScopePulley6/8
  PS>Sim1/2(Out2) -> ScopePulley6/2
  PS>Sim1/3(Out3) -> ScopePulley6/3
  PS>Sim1/6(Out6) -> ScopePulley6/6
  Constant/1 -> Divide/2
  Divide/1 -> [PinLoad_R_tonne]
  Demux/2 -> Gain1/1
  Gain1/1 -> Divide/1
  connections:
  WireB/RConn1 -- Pulley 6/RConn2
  Sheave6/RConn1 -- Pulley 6/LConn1
  Pulley 6/RConn1 -- WireA/RConn1
  Revolute Pulley6/LConn1 -- Conn2/RConn1 -- " "/LConn1 -- " 4"/LConn1
  PS>Sim1/LConn2 -- Revolute Pulley6/RConn3 -- w (rad/s)1/LConn1
  Revolute Pulley6/RConn4 -- PS>Sim1/LConn3
  " "/RConn1 -- right face/RConn1
  Sheave6/LConn1 -- Revolute Pulley6/RConn1
  Revolute Pulley6/RConn2 -- PS>Sim1/LConn1
  Revolute Pulley6/RConn5 -- PS>Sim1/LConn4
  Revolute Pulley6/RConn9 -- PS>Sim1/LConn8
  Revolute Pulley6/RConn8 -- PS>Sim1/LConn7
  " 4"/RConn1 -- left face/RConn1
  Revolute Pulley6/RConn6 -- PS>Sim1/LConn5
  Revolute Pulley6/RConn7 -- PS>Sim1/LConn6
  Nm/RConn1 -- Revolute Pulley6/LConn2
